simulink model "Practica22 "  (R2024b)
settings: Solver=VariableStepAuto  StartTime=0.0  StopTime=30  RelTol=1e-3
libraries: slpidlib x1
settings DataIOCC: ReturnWorkspaceOutputs=off  TimeSaveName=t
settings DebuggingCC: AlgebraicLoopMsg=none  ArtificialAlgebraicLoopMsg=none  MaxConsecutiveZCsMsg=none  OperatingPointInterfaceChecksumMismatchMsg=none

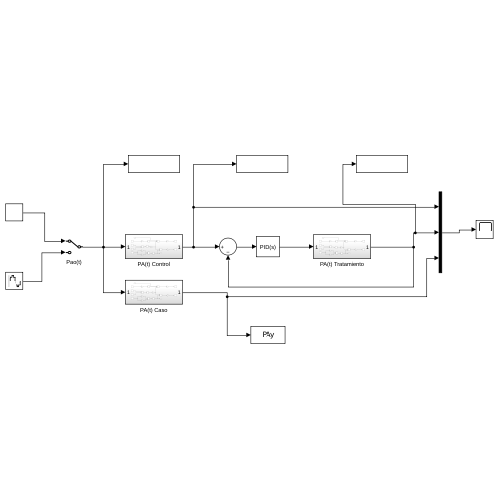
[thumbnail: Simulink's stored preview of the top-level diagram]
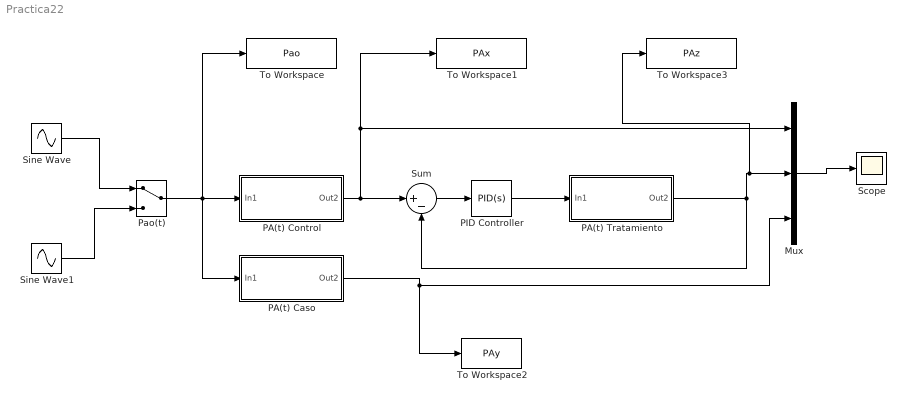
== system Practica22  ==
  Mux : Mux  Inputs=3
  PA(t) Caso : Subsystem
  PA(t) Control : Subsystem
  PA(t) Tratamiento : Subsystem
  PID Controller : slpidlib/PID Controller  Controller=PID  Form=Parallel  TimeDomain=Continuous-time  UseExternalTs=off  SampleTime=-1  IntegratorMethod=Forward Euler  FilterMethod=Forward Euler  ControllerParametersSource=internal  P=254.794522788379  I=4952.03786900602  UseKiTs=off  D=1.23977039590424  UseExternalDerivativeSource=off  N=26057.2692515696  UseFilter=on  TunerSelectOption=Transfer Function Based (PID Tuner App)  InitialConditionSource=internal  InitialConditionForIntegrator=0  InitialConditionForFilter=0  DifferentiatorICPrevScaledInput=0  ExternalReset=none  TrackingMode=off  Kt=1  LimitOutput=off  SatLimitsSource=internal  UpperSaturationLimit=inf  LowerSaturationLimit=-inf  LinearizeAsGain=on  AntiWindupMode=none  Kb=1  LimitIntegrator=off  UpperIntegratorSaturationLimit=inf  LowerIntegratorSaturationLimit=-inf  POutMin=[]  POutMax=[]  IOutMin=[]  IOutMax=[]  DOutMin=[]  DOutMax=[]  NOutMin=[]  NOutMax=[]  SumOutMin=[]  SumOutMax=[]  SaturationOutMin=[]  SaturationOutMax=[]  PParamMin=[]  PParamMax=[]  IParamMin=[]  IParamMax=[]  DParamMin=[]  DParamMax=[]  NParamMin=[]  NParamMax=[]  KbParamMin=[]  KbParamMax=[]  KtParamMin=[]  KtParamMax=[]  KbOutMin=[]  KbOutMax=[]  KtOutMin=[]  KtOutMax=[]  IntegratorOutMin=[]  IntegratorOutMax=[]  FilterOutMin=[]  FilterOutMax=[]  SumI1OutMin=[]  SumI1OutMax=[]  SumI2OutMin=[]  SumI2OutMax=[]  SumI3OutMin=[]  SumI3OutMax=[]  SumI4OutMin=[]  SumI4OutMax=[]  SumDOutMin=[]  SumDOutMax=[]  DifferentiatorOutMin=[]  DifferentiatorOutMax=[]  FilterDiffOutCoefMin=[]  FilterDiffOutCoefMax=[]  ReciprocalOutMin=[]  ReciprocalOutMax=[]  SumDenOutMin=[]  SumDenOutMax=[]  SumNumOutMin=[]  SumNumOutMax=[]  DivideOutMin=[]  DivideOutMax=[]  UdiffTsProdOutMin=[]  UdiffTsProdOutMax=[]  NTsProdOutMin=[]  NTsProdOutMax=[]  UintegralTsProdOutMin=[]  UintegralTsProdOutMax=[]  UngainTsProdOutMin=[]  UngainTsProdOutMax=[]  ClampingZeroOutDataTypeStr=Inherit: Inherit via back propagation  ClampingZeroOutMin=[]  ClampingZeroOutMax=[]  FilterDenConstantOutDataTypeStr=Inherit: Inherit via back propagation  FilterDenConstantOutMin=[]  FilterDenConstantOutMax=[]  PCopyOutDataTypeStr=Inherit: Inherit via back propagation  PCopyOutMin=[]  PCopyOutMax=[]  NCopyOutDataTypeStr=Inherit: Inherit via back propagation  NCopyOutMin=[]  NCopyOutMax=[]  IntegratorContinuousStateAttributes=''  IntegratorStateMustResolveToSignalObject=off  IntegratorRTWStateStorageClass=Auto  FilterContinuousStateAttributes=''  FilterStateMustResolveToSignalObject=off  FilterRTWStateStorageClass=Auto  ParallelPVariant=InternalParameters  IdealPVariant=Disabled  IVariant=InternalParameters  DVariant=InternalParameters  IntegratorVariant=Continuous  SatVariant=Disabled  AWVariant=Passthrough  PCopyVariant=Disabled  TRVariant=Disabled  FdbkBlocksVariant=Forward  IdealPFdbkVariant=Disabled  SatFdbkVariant=Disabled  DerivativeFilterVariant=ContFilter  NVariant=InternalParameters  NCopyVariant=Disabled  FilterICVariant=InternalICsFilter  IntegratorICVariant=InternalICs  ExternalResetVariant=Disabled  TRSumVariant=Passthrough  SumFdbkVariant=Disabled  SumVariant=Sum_PID  TsampFilterVariant=InternalTs  TsampNgainVariant=Passthrough  TsampIntegralVariant=Disabled_SignalSpec  ExternalSaturationOutDataTypeStr=Inherit: Same as second input  DerivativeSourceVariant=ErrorSignal  PreIntVariant=InternalPreInt
  Pao(t) : ManualSwitch
  Scope : Scope
  Sine Wave : Sin  Amplitude=2.5  Frequency=pi/2  SampleTime=0.1
  Sine Wave1 : Sin  Amplitude=2.5  Frequency=pi  SampleTime=0.1
  Sum : Sum  Inputs=|+-
  To Workspace : ToWorkspace  VariableName=Pao  SampleTime=-1
  To Workspace1 : ToWorkspace  VariableName=PAx  SampleTime=-1
      settings: Save2DSignal=2-D array (concatenate along first dimension)
  To Workspace2 : ToWorkspace  VariableName=PAy  SampleTime=-1
      settings: Save2DSignal=2-D array (concatenate along first dimension)
  To Workspace3 : ToWorkspace  VariableName=PAz  SampleTime=-1
      settings: Save2DSignal=2-D array (concatenate along first dimension)
  wires:
  Sine Wave/1 -> Pao(t)/1
  Sine Wave1/1 -> Pao(t)/2
  Pao(t)/1 -> PA(t) Caso/1(In1), To Workspace/1, PA(t) Control/1(In1)
  Sum/1 -> PID Controller/1
  PA(t) Tratamiento/1(Out2) -> To Workspace3/1, Mux/2, Sum/2
  PA(t) Control/1(Out2) -> Mux/1, To Workspace1/1, Sum/1
  PA(t) Caso/1(Out2) -> Mux/3, To Workspace2/1
  Mux/1 -> Scope/1
  PID Controller/1 -> PA(t) Tratamiento/1(In1)

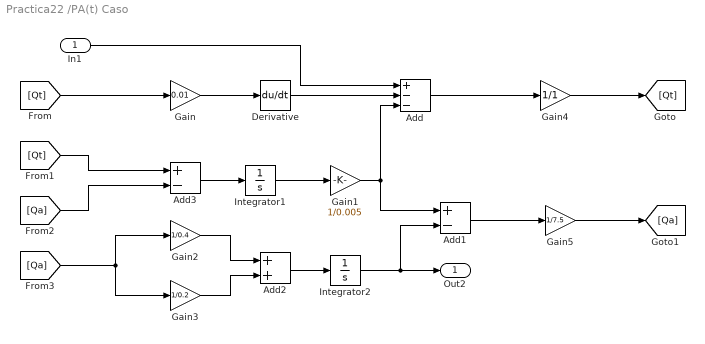
== system Practica22 /PA(t) Caso ==
  In1 : Inport
  Add : Sum  Inputs=+--
  Add1 : Sum  Inputs=+-
  Add2 : Sum
  Add3 : Sum  Inputs=+-
  Derivative : Derivative
  Gain : Gain  Gain=0.01
  Gain1 : Gain  Gain=1/0.005
  Gain2 : Gain  Gain=1/0.4
  Gain3 : Gain  Gain=1/0.2
  Gain4 : Gain  Gain=1/1
  Gain5 : Gain  Gain=1/7.5
  Integrator1 : Integrator
  Integrator2 : Integrator
  Out2 : Outport
  wires:
  [Qt] -> Gain/1
  Gain/1 -> Derivative/1
  Add/1 -> Gain4/1
  [Qa] -> Gain3/1, Gain2/1
  Integrator2/1 -> Out2/1, Add1/2
  Derivative/1 -> Add/2
  Add1/1 -> Gain5/1
  [Qt] -> Add3/1
  Gain2/1 -> Add2/1
  In1/1 -> Add/1
  [Qa] -> Add3/2
  Gain4/1 -> [Qt]
  Add2/1 -> Integrator2/1
  Gain3/1 -> Add2/2
  Gain5/1 -> [Qa]
  Gain1/1 -> Add1/1, Add/3
  Integrator1/1 -> Gain1/1
  Add3/1 -> Integrator1/1

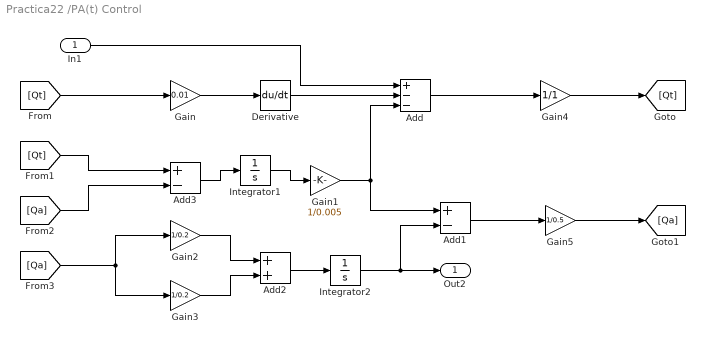
== system Practica22 /PA(t) Control ==
  In1 : Inport
  Add : Sum  Inputs=+--
  Add1 : Sum  Inputs=+-
  Add2 : Sum
  Add3 : Sum  Inputs=+-
  Derivative : Derivative
  Gain : Gain  Gain=0.01
  Gain1 : Gain  Gain=1/0.005
  Gain2 : Gain  Gain=1/0.2
  Gain3 : Gain  Gain=1/0.2
  Gain4 : Gain  Gain=1/1
  Gain5 : Gain  Gain=1/0.5
  Integrator1 : Integrator
  Integrator2 : Integrator
  Out2 : Outport
  wires:
  [Qt] -> Gain/1
  Gain/1 -> Derivative/1
  In1/1 -> Add/1
  Derivative/1 -> Add/2
  [Qt] -> Add3/1
  [Qa] -> Add3/2
  [Qa] -> Gain3/1, Gain2/1
  Gain3/1 -> Add2/2
  Gain2/1 -> Add2/1
  Add2/1 -> Integrator2/1
  Integrator2/1 -> Out2/1, Add1/2
  Add1/1 -> Gain5/1
  Add/1 -> Gain4/1
  Gain4/1 -> [Qt]
  Gain5/1 -> [Qa]
  Add3/1 -> Integrator1/1
  Integrator1/1 -> Gain1/1
  Gain1/1 -> Add1/1, Add/3

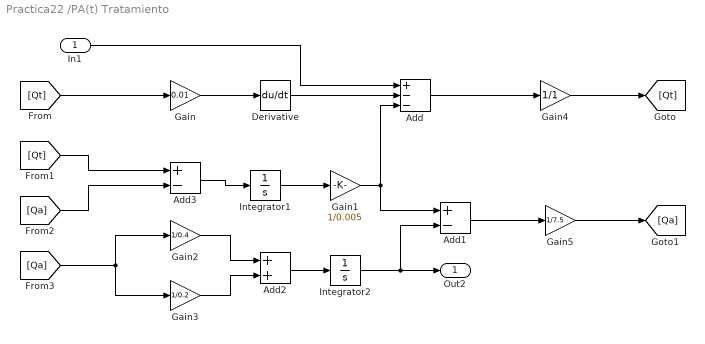
== system Practica22 /PA(t) Tratamiento ==
  In1 : Inport
  Add : Sum  Inputs=+--
  Add1 : Sum  Inputs=+-
  Add2 : Sum
  Add3 : Sum  Inputs=+-
  Derivative : Derivative
  Gain : Gain  Gain=0.01
  Gain1 : Gain  Gain=1/0.005
  Gain2 : Gain  Gain=1/0.4
  Gain3 : Gain  Gain=1/0.2
  Gain4 : Gain  Gain=1/1
  Gain5 : Gain  Gain=1/7.5
  Integrator1 : Integrator
  Integrator2 : Integrator
  Out2 : Outport
  wires:
  [Qt] -> Gain/1
  Integrator2/1 -> Out2/1, Add1/2
  Derivative/1 -> Add/2
  Gain2/1 -> Add2/1
  Gain3/1 -> Add2/2
  [Qa] -> Add3/2
  [Qt] -> Add3/1
  Gain4/1 -> [Qt]
  Gain5/1 -> [Qa]
  Add2/1 -> Integrator2/1
  [Qa] -> Gain3/1, Gain2/1
  In1/1 -> Add/1
  Gain/1 -> Derivative/1
  Add1/1 -> Gain5/1
  Add/1 -> Gain4/1
  Add3/1 -> Integrator1/1
  Integrator1/1 -> Gain1/1
  Gain1/1 -> Add1/1, Add/3
